simulink model "drone2"  (R2022b)
settings: Solver=VariableStepAuto  StartTime=0.0  StopTime=10.0  RelTol=1e-3
settings Model: Creator=depressedcoder  LastModifiedBy=depressedcoder

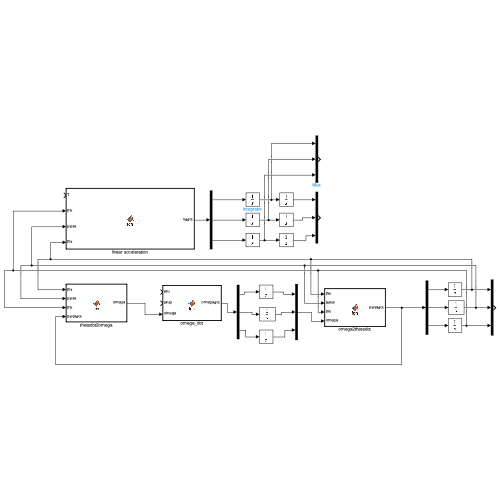
[thumbnail: Simulink's stored preview of the top-level diagram]
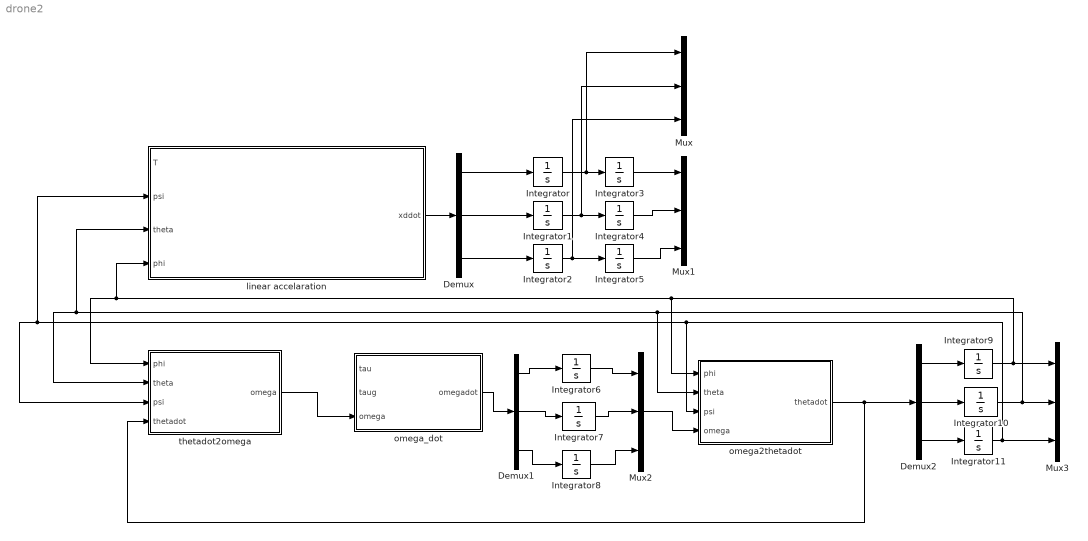
== system drone2 ==
  Demux : Demux  Outputs=3
  Demux1 : Demux  Outputs=3
  Demux2 : Demux  Outputs=3
  Integrator{,1..11} (12 alike) : Integrator
  Mux{,1..3} (4 alike) : Mux  Inputs=3
  linear accelaration : MATLAB Function  TreatAsAtomicUnit=on
  omega2thetadot : MATLAB Function  TreatAsAtomicUnit=on
  omega_dot : MATLAB Function  TreatAsAtomicUnit=on
  thetadot2omega : MATLAB Function  TreatAsAtomicUnit=on
  wires:
  linear accelaration/1(xddot) -> Demux/1
  Demux/1 -> Integrator/1
  Demux/2 -> Integrator1/1
  Demux/3 -> Integrator2/1
  Integrator/1 -> Mux/1, Integrator3/1
  Integrator1/1 -> Mux/2, Integrator4/1
  Integrator2/1 -> Mux/3, Integrator5/1
  Integrator3/1 -> Mux1/1
  Integrator4/1 -> Mux1/2
  Integrator5/1 -> Mux1/3
  omega_dot/1(omegadot) -> Demux1/1
  Demux1/1 -> Integrator6/1
  Demux1/2 -> Integrator7/1
  Demux1/3 -> Integrator8/1
  Integrator6/1 -> Mux2/1
  Integrator7/1 -> Mux2/2
  Integrator8/1 -> Mux2/3
  thetadot2omega/1(omega) -> omega_dot/3(omega)
  Mux2/1 -> omega2thetadot/4(omega)
  omega2thetadot/1(thetadot) -> thetadot2omega/4(thetadot), Demux2/1
  Integrator11/1 -> linear accelaration/2(psi), thetadot2omega/3(psi), omega2thetadot/3(psi), Mux3/3
  Integrator10/1 -> omega2thetadot/2(theta), linear accelaration/3(theta), thetadot2omega/2(theta), Mux3/2
  Integrator9/1 -> linear accelaration/4(phi), thetadot2omega/1(phi), omega2thetadot/1(phi), Mux3/1
  Demux2/3 -> Integrator11/1
  Demux2/2 -> Integrator10/1
  Demux2/1 -> Integrator9/1

== matlab function drone2/omega_dot ==
  data: tau input; taug input; omegadot output; omega input
function omegadot = fcn(tau,taug,omega)
I = diag([2.3951,2.3951,3.2347]*10^-5);
omegadot = inv(I)*(tau - cross(omega,I*omega) - taug);

== matlab function drone2/linear accelaration ==
  data: T input; xddot output; psi input; theta input; phi input
function xddot = fcn(T,psi,theta,phi)

xddot = [0.0 ; 0.0 ; 0.0] ;
m = 34*10^-3 ;
g = 9.8 ;
F_x_g = 0.0;
F_y_g = 0.0;

xddot(1,1) = (T/m)*(sin(psi)*sin(phi) + cos(psi)*cos(phi)*sin(theta)) - (F_x_g/m);
xddot(2,1) = (T/m)*(-cos(psi)*sin(phi) + sin(psi)*cos(phi)*sin(theta)) - (F_y_g/m);
xddot(3,1) = (T/m)*(cos(psi)*cos(theta)) - g;

== matlab function drone2/thetadot2omega ==
  data: phi input; omega output; theta input; psi input; thetadot input
function omega = fcn(phi,theta,psi,thetadot)
R = [1 0 -sin(theta) ; 0 cos(phi) cos(theta)*sin(phi) ; 0 -sin(phi) cos(theta)*cos(phi)] ;
omega = R*thetadot;

== matlab function drone2/omega2thetadot ==
  data: phi input; thetadot output; theta input; psi input; omega input
function thetadot = fcn(phi,theta,psi,omega)
R = inv([1 0 -sin(theta) ; 0 cos(phi) cos(theta)*sin(phi) ; 0 -sin(phi) cos(theta)*cos(phi)]) ;
thetadot = R*omega;
